simulink library "iq_splitter_8c4r_lib"  (Simulink 8.7)
settings: Solver=ode45  StartTime=0.0  StopTime=10.0  RelTol=1e-3
undefined symbols (not defined in the file): AdvDSPBChannelOutDisplay, dpoly, dspba_ChannelInVis, dspba_ChannelOutVis, dspba_internal_get_channel_ports, dspba_internal_get_demux_ports, latency, value
libraries: DSPBAPrim x9, Pipereg_lib x2, DSPBABase x1
settings Model: Creator=bigcat  LastModifiedBy=5g

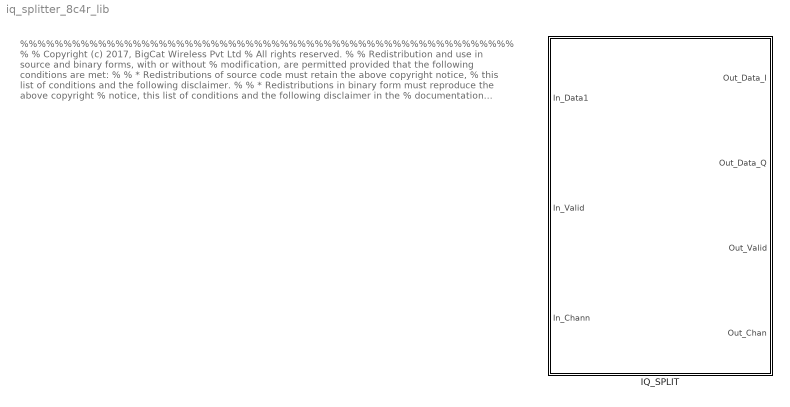
== system iq_splitter_8c4r_lib ==
  note: %%%%%%%%%%%%%%%%%%%%%%%%%%%%%%%%%%%%%%%%%%%%%%%%%%%%%%%%%
      |  %
      |  % Copyright (c) 2017, BigCat Wireless Pvt Ltd
      |  % All rights reserved.
      |  %
      |  % Redistribution and use in source and binary forms, with or without
      |  % modification, are permitted provided that the following conditions are met:
      |  %
      |  %     * Redistributions of source code must retain the above copyright notice,
      |  %       this list of conditions and the following disclaimer.
      |  %
      |  %     * Redistributions in binary form must reproduce the above copyright
      |  %       notice, this list of conditions and the following disclaimer in the
      |  %       documentation and/or other materials provided with the distribution.
      |  %
      |  %     * Neither the name of the copyright holder nor the names of its contributors
      |  %       may be used to endorse or promote products derived from this software
      |  %       without specific prior written permission.
      |  %
      |  %
      |  %
      |  % THIS SOFTWARE IS PROVIDED BY THE COPYRIGHT HOLDERS AND CONTRIBUTORS "AS IS"
      |  % AND ANY EXPRESS OR IMPLIED WARRANTIES, INCLUDING, BUT NOT LIMITED TO, THE
      |  % IMPLIED WARRANTIES OF MERCHANTABILITY AND FITNESS FOR A PARTICULAR PURPOSE ARE
      |  % DISCLAIMED. IN NO EVENT SHALL THE COPYRIGHT HOLDER OR CONTRIBUTORS BE LIABLE
      |  % FOR ANY DIRECT, INDIRECT, INCIDENTAL, SPECIAL, EXEMPLARY, OR CONSEQUENTIAL
      |  % DAMAGES (INCLUDING, BUT NOT LIMITED TO, PROCUREMENT OF SUBSTITUTE GOODS OR
      |  % SERVICES; LOSS OF USE, DATA, OR PROFITS; OR BUSINESS INTERRUPTION) HOWEVER
      |  % CAUSED AND ON ANY THEORY OF LIABILITY, WHETHER IN CONTRACT, STRICT LIABILITY,
      |  % OR TORT (INCLUDING NEGLIGENCE OR OTHERWISE) ARISING IN ANY WAY OUT OF THE USE
      |  % OF THIS SOFTWARE, EVEN IF ADVISED OF THE POSSIBILITY OF SUCH DAMAGE.
      |  %
      |   %%%%%%%%%%%%%%%%%%%%%%%%%%%%%%%%%%%%%%%%%%%%%%%%%%%%%%%%%%
  IQ_SPLIT : Subsystem  mask{Latency=0, ClockMargin=0, Pipeline_stages=0}
      mask Display:
      | disp('IQ_SPLITTER');
      | port_label('input',1,'d');
      | port_label('input',2,'v');
      | port_label('input',3,'c');
      | port_label('output',1,'q_I');
      | port_label('output',2,'q_Q');
      | port_label('output',3,'q_v');
      | port_label('output',4,'q_c');

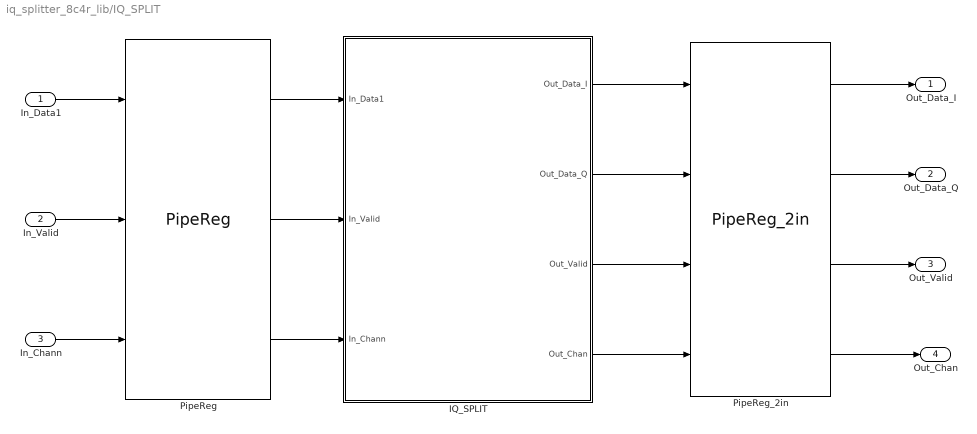
== system iq_splitter_8c4r_lib/IQ_SPLIT ==
  In_Data1 : Inport
  In_Valid : Inport  Port=2
  In_Chann : Inport  Port=3
  IQ_SPLIT : Subsystem
  PipeReg : Pipereg_lib/PipeReg  NPipe=Pipeline_stages  Clock_Margin=ClockMargin
  PipeReg_2in : Pipereg_lib/PipeReg_2in  NPipe=Pipeline_stages  Clock_Margin=ClockMargin
  Out_Data_I : Outport
  Out_Data_Q : Outport  Port=2
  Out_Valid : Outport  Port=3
  Out_Chan : Outport  Port=4
  wires:
  PipeReg/1 -> IQ_SPLIT/1(In_Data1)
  PipeReg/2 -> IQ_SPLIT/2(In_Valid)
  PipeReg/3 -> IQ_SPLIT/3(In_Chann)
  In_Data1/1 -> PipeReg/1
  In_Valid/1 -> PipeReg/2
  In_Chann/1 -> PipeReg/3
  IQ_SPLIT/2(Out_Data_Q) -> PipeReg_2in/2
  IQ_SPLIT/1(Out_Data_I) -> PipeReg_2in/1
  IQ_SPLIT/3(Out_Valid) -> PipeReg_2in/3
  IQ_SPLIT/4(Out_Chan) -> PipeReg_2in/4
  PipeReg_2in/1 -> Out_Data_I/1
  PipeReg_2in/2 -> Out_Data_Q/1
  PipeReg_2in/3 -> Out_Valid/1
  PipeReg_2in/4 -> Out_Chan/1

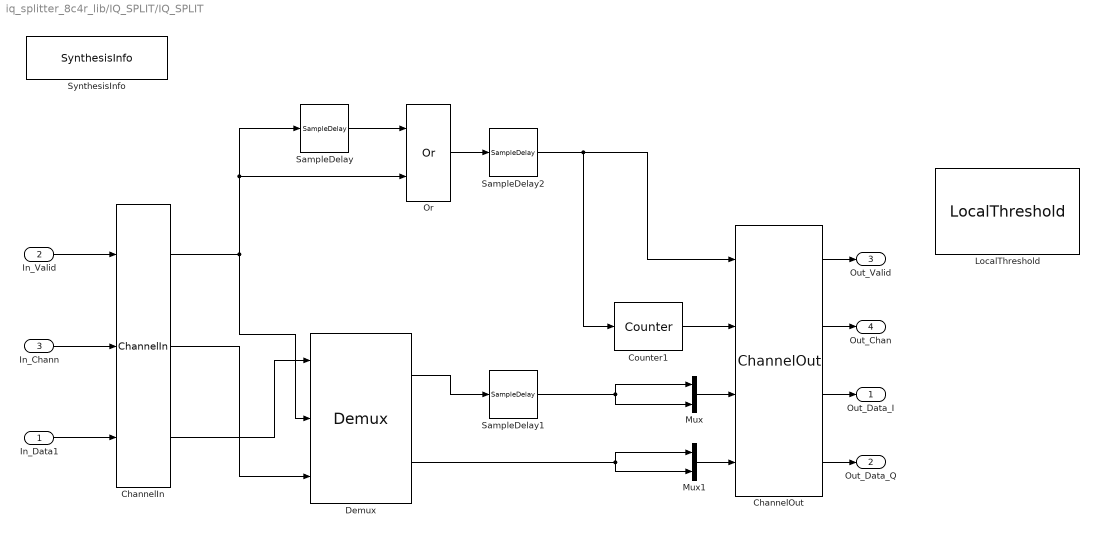
== system iq_splitter_8c4r_lib/IQ_SPLIT/IQ_SPLIT ==
  In_Data1 : Inport
  In_Valid : Inport  Port=2
  In_Chann : Inport  Port=3
  ChannelIn : DSPBAPrim/ChannelIn  primtype=channelin  nInputs=dspba_internal_get_channel_ports(gcb)  nOutputs=dspba_internal_get_channel_ports(gcb)  omode=Inherit via internal rule  otype=sfix(16)  scale=2^-15  rndmethod=Unbiased  factor=1  satmethod=Symmetric  shift_vec=[0 1 2 -1]  value=1  inPortNames=['v'; 'c'; '0'; '1'; '2'; '3'; '4'; '5'; '6'; '7'; '8'; '9'; 'A'; 'B'; 'D'; 'E'; 'F'; 'G'; 'H'; 'I'; 'J'; 'K'; 'L'; 'M'; 'N'; 'O'; 'P'; 'Q'; 'R'; 'S'; 'T'; 'U'; 'W'; 'X'; 'Y'; 'Z']  outPortNames=['v'; 'c'; '0'; '1'; '2'; '3'; '4'; '5'; '6'; '7'; '8'; '9'; 'A'; 'B'; 'D'; 'E'; 'F'; 'G'; 'H'; 'I'; 'J'; 'K'; 'L'; 'M'; 'N'; 'O'; 'P'; 'Q'; 'R'; 'S'; 'T'; 'U'; 'W'; 'X'; 'Y'; 'Z']  dspbaimage=dspba_prim.jpg  text=fprintf('In');  style=Optimised  dataSignals=1  foldingEnabled=off  channels=1  sampleRate=200  packetBeginPresent=off  packetBeginEnabled=off  visibilities=dspba_ChannelInVis(gcb)  latencyCorrection=0  version=20141013
  ChannelOut : DSPBAPrim/ChannelOut  primtype=channelout  nInputs=dspba_internal_get_channel_ports(gcb)  nOutputs=dspba_internal_get_channel_ports(gcb)  omode=Inherit via internal rule  otype=sfix(16)  scale=2^-15  rndmethod=Unbiased  factor=1  satmethod=Symmetric  shift_vec=[0 1 2 -1]  value=2  inPortNames=['v'; 'c'; '0'; '1'; '2'; '3'; '4'; '5'; '6'; '7'; '8'; '9'; 'A'; 'B'; 'D'; 'E'; 'F'; 'G'; 'H'; 'I'; 'J'; 'K'; 'L'; 'M'; 'N'; 'O'; 'P'; 'Q'; 'R'; 'S'; 'T'; 'U'; 'W'; 'X'; 'Y'; 'Z']  outPortNames=['v'; 'c'; '0'; '1'; '2'; '3'; '4'; '5'; '6'; '7'; '8'; '9'; 'A'; 'B'; 'D'; 'E'; 'F'; 'G'; 'H'; 'I'; 'J'; 'K'; 'L'; 'M'; 'N'; 'O'; 'P'; 'Q'; 'R'; 'S'; 'T'; 'U'; 'W'; 'X'; 'Y'; 'Z']  dspbaimage=dspba_prim.jpg  text=fprintf('Out%s', AdvDSPBChannelOutDisplay(latency));  style=Optimised  dataSignals=2  foldingEnabled=off  channels=1  sampleRate=200  packetBeginPresent=off  packetBeginEnabled=off  visibilities=dspba_ChannelOutVis(gcb)  latency=2  latencyCorrection=0  version=20141013
  Counter1 : DSPBAPrim/Counter  primtype=counter  nInputs=1  nOutputs=1  omode=Inherit via internal rule  otype=ufix(16)  scale=2^-0  rndmethod=Unbiased  factor=1  satmethod=Symmetric  shift_vec=[0 1 2 -1]  value=[3 4 1]  inPortNames=[' '; ' ';]  outPortNames=[' ']  dspbaimage=dspba_prim.jpg  text=fprintf('counter\n[%d %d %d]', value(1), value(2), value(3));  style=Optimised  visibilities=8 + 1024  version=20090407
  Demux : DSPBAPrim/Demux  primtype=demux  nInputs=3  nOutputs=dspba_internal_get_demux_ports(gcb)  omode=Inherit via internal rule  otype=sfix(16)  scale=2^-15  rndmethod=Unbiased  factor=1  satmethod=Symmetric  shift_vec=[0 1]  value=2  inPortNames=['q'; 'v'; 'c']  outPortNames=['c0'; 'c1']  dspbaimage=dspba_prim.jpg  text=fprintf('demux');  style=Optimised  visibilities=1536  version=20100120
  LocalThreshold : DSPBABase/LocalThreshold  margin=ClockMargin  delayRegOrRAMThresholdBits=10000  MediumDualMemThresholdBits=10000  LargeDualMemThresholdBits=-1  hardMultiplierThresholdLuts=-1  version=0
  Mux : Mux  Inputs=2
  Mux1 : Mux  Inputs=2
  Or : DSPBAPrim/Or  primtype=or  nInputs=2  nOutputs=1  omode=Inherit via internal rule  otype=sfix(16)  scale=2^-15  rndmethod=Unbiased  factor=1  satmethod=Symmetric  shift_vec=[0 1 2 -1]  value=0  inPortNames=[' '; ' '; ' '; ' '; ' '; ' '; ' '; ' '; ' '; ' '; ' '; ' '; ' '; ' '; ' '; ' '; ]  outPortNames=[' ']  dspbaimage=dspba_prim.jpg  text=fprintf('|');  style=Optimised  visibilities=8+2  version=20090407
  SampleDelay : DSPBAPrim/SampleDelay  primtype=sampdelay  nInputs=1  nOutputs=1  omode=Inherit via internal rule  otype=sfix(16)  scale=2^-15  rndmethod=Unbiased  factor=1  satmethod=Symmetric  shift_vec=[0 1 2 -1]  value=2  inPortNames=[' '; ' ';]  outPortNames=[' ']  dspbaimage=dspba_prim.jpg  text=dpoly(1, eye(1,value+1), 'z')  style=Optimised  visibilities=8 + 1024 + 2^17 + 2^18  flexible=off  slackgroup=0  augmented=0  version=20090407  advOptions=[]
  SampleDelay1 : DSPBAPrim/SampleDelay  primtype=sampdelay  nInputs=1  nOutputs=1  omode=Inherit via internal rule  otype=sfix(16)  scale=2^-15  rndmethod=Unbiased  factor=1  satmethod=Symmetric  shift_vec=[0 1 2 -1]  value=1  inPortNames=[' '; ' ';]  outPortNames=[' ']  dspbaimage=dspba_prim.jpg  text=dpoly(1, eye(1,value+1), 'z')  style=Optimised  visibilities=8 + 1024 + 2^17 + 2^18  flexible=off  slackgroup=0  augmented=0  version=20090407  advOptions=[]
  SampleDelay2 : DSPBAPrim/SampleDelay  primtype=sampdelay  nInputs=1  nOutputs=1  omode=Inherit via internal rule  otype=sfix(16)  scale=2^-15  rndmethod=Unbiased  factor=1  satmethod=Symmetric  shift_vec=[0 1 2 -1]  value=1  inPortNames=[' '; ' ';]  outPortNames=[' ']  dspbaimage=dspba_prim.jpg  text=dpoly(1, eye(1,value+1), 'z')  style=Optimised  visibilities=8 + 1024 + 2^17 + 2^18  flexible=off  slackgroup=0  augmented=0  version=20090407  advOptions=[]
  SynthesisInfo : DSPBAPrim/SynthesisInfo  primtype=synthinfo  nInputs=0  nOutputs=0  omode=Inherit via internal rule  otype=sfix(16)  scale=2^-15  rndmethod=Truncate  factor=1  satmethod=Symmetric  shift_vec=[0 1 2 -1]  value=99  inPortNames=[' '; ' ';]  outPortNames=[' ']  dspbaimage=dspba_prim_ctrl.jpg  text=fprintf('Style=%s', style);  style=Scheduled  visibilities=2^15+2^17+2^18+2^19  constraintInUse=on  constraintRelation==  constraintLimit=Latency  bitAccurate=off  version=20090407
  Out_Data_I : Outport
  Out_Data_Q : Outport  Port=2
  Out_Valid : Outport  Port=3
  Out_Chan : Outport  Port=4
  wires:
  In_Data1/1 -> ChannelIn/3
  ChannelOut/3 -> Out_Data_I/1
  In_Chann/1 -> ChannelIn/2
  In_Valid/1 -> ChannelIn/1
  ChannelOut/1 -> Out_Valid/1
  ChannelOut/2 -> Out_Chan/1
  ChannelIn/1 -> Demux/2, Or/2, SampleDelay/1
  ChannelIn/2 -> Demux/3
  ChannelIn/3 -> Demux/1
  ChannelOut/4 -> Out_Data_Q/1
  Demux/1 -> SampleDelay1/1
  SampleDelay/1 -> Or/1
  Or/1 -> SampleDelay2/1
  SampleDelay2/1 -> Counter1/1, ChannelOut/1
  Counter1/1 -> ChannelOut/2
  Mux/1 -> ChannelOut/3
  SampleDelay1/1 -> Mux/1, Mux/2
  Mux1/1 -> ChannelOut/4
  Demux/2 -> Mux1/2, Mux1/1
